simulink model "LinLongNormal_Aquila_Claws_Discrete"  (R2017a)
settings: Solver=VariableStepAuto  StartTime=0.0  StopTime=500  RelTol=1e-3  EnableMultiTasking=on
model workspace: external: MAT-File (data not in the file)
undefined symbols (not defined in the file): AP_AltLoop_AltCmdLPFDenTau, AP_AltLoop_altRateCmdMaxLimMps, AP_AltLoop_altRateCmdMinLimMps, AP_AltLoop_Kd, AP_AltLoop_Ki, AP_AltLoop_Ki_WindupMaxLim, AP_AltLoop_Ki_WindupMinLim, AP_AltLoop_Kp, AP_ClimbRate_LPFDenTau, AP_ClimbRateLoop_ClimbRateCmdLPFDenTau, AP_ClimbRateLoop_Ki, AP_ClimbRateLoop_Kp, AP_ClimbRateLoop_LLFiltDenCoe, AP_ClimbRateLoop_LLFiltNumCoe, AP_ClimbRateLoop_MaxPitchCmdrad, AP_ClimbRateLoop_MinPitchCmdrad, AP_FlexLoop_NotchDampingDen, AP_FlexLoop_NotchDampingNum, AP_FlexLoop_NotchFreq, AP_FlexLoop_nzFdbk_Kp, AP_FlexLoop_nzFdbkLLFiltDenCoe, AP_FlexLoop_nzFdbkLLFiltNumCoe, AP_FlexLoop_wn_ElvRollOff, AP_GLALoop_MaxSplCmdDeg, AP_GLALoop_MinSplCmdDeg, AP_GLALoop_nzFdbk_Ki, AP_GLALoop_nzFdbk_Kp, AP_GLALoop_nzFdbkDenTau, AP_GndTrkLoop_CmdLPFDenTau, AP_GndTrkLoop_Kd, AP_GndTrkLoop_Kp, AP_GndTrkLoop_phiCmdMaxLimDeg, AP_GndTrkLoop_phiCmdMinLimDeg, AP_GndTrkLoop_phiRateCmdMaxLimDps, AP_GndTrkLoop_phiRateCmdMinLimDps, AP_PitchLoop_DerivLPFDenTau, AP_PitchLoop_Kd, AP_PitchLoop_Kff, AP_PitchLoop_Ki, AP_PitchLoop_Kp, AP_PitchLoop_Kq, AP_PitchLoop_Notch1BWfactor, AP_PitchLoop_Notch1CosFreqNorm, AP_PitchLoop_qFdbkLFLLFiltDenCoe, AP_PitchLoop_qFdbkLFLLFiltNumCoe, AP_PitchLoop_qFdbkLLFiltDenCoe, AP_PitchLoop_qFdbkLLFiltNumCoe, AP_PitchLoop_thetaCmdLPFDenTau, AP_PitchLoop_wn_ElvRollOff, AP_PitchLoop_zeta_ElvRollOff, AP_PwrLoop_ClimbRateCmdLPFDenTau, AP_PwrLoop_Ki, AP_PwrLoop_Kp, AP_PwrLoop_Kvadv, AP_PwrLoop_LLFiltDenCoe, AP_PwrLoop_LLFiltNumCoe, AP_PwrLoop_MaxThrCmdNorm, AP_PwrLoop_MinThrCmdNorm, AP_PwrLoop_wn_ThrRollOff, AP_PwrLoop_zeta_ThrRollOff ... (+59)
libraries: discretizing x18, aerolibconvert2 x15, simulink x10, Washout x1, cstblocks x1
(part 1 of 2)
settings Model: Creator=The MathWorks, Inc.  LastModifiedBy=hbolandhemmat
settings DataIOCC: LimitDataPoints=on
settings OptimizationCC: LifeSpan=inf
settings DebuggingCC: AllowSymbolicDim=off  SFUnexpectedBacktrackingDiag=warning  SFNoUnconditionalDefaultTransitionDiag=warning  SFExecutionAtInitializationDiag=none
settings ModelReferenceCC: PropagateSignalLabelsOutOfModel=off
settings GRTTargetCC: TargetLangStandard=C89/C90 (ANSI)
settings ConfigComp: CovMetricSettings=dw  CovHtmlReporting=on  CovSaveCumulativeToWorkspaceVar=on  CovSaveSingleToWorkspaceVar=on  CovExternalEMLEnable=off

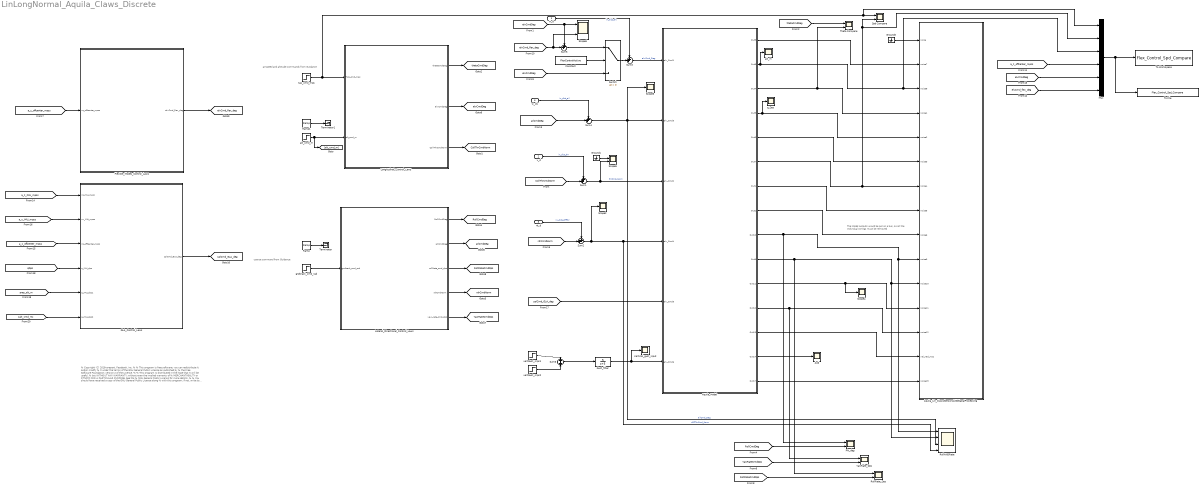
== system LinLongNormal_Aquila_Claws_Discrete ==
  note: coarse command from Guidance
  note: The Model outputs would be put on a bus, so all
      | the individual strings must be removed
  note: airspeed and altitude commands
      | from Guidance
  note: % Copyright (C) 2018-present, Facebook, Inc.
      | %
      | % This program is free software; you can redistribute it and/or modify
      | % it under the terms of the GNU General Public License as published by
      | % the Free Software Foundation; version 2 of the License.
      | %
      | % This program is distributed in the hope that it will be useful,
      | % but WITHOUT ANY WARRANTY; without even the implied warranty of
      | % MERCHANTABILITY or FITNESS FOR A PARTICULAR PURPOSE. See the
      | % GNU General Public License for more details.
      | %
      | % You should have received a copy of the GNU General Public License along
      | % with this program; if not, write to the Free Software Foundation, Inc.,
      | % 51 Franklin Street, Fifth Floor, Boston, MA 02110-1301 USA.
  w_d : Inport
  v_d : Inport  Port=2
  nt_d : Inport  Port=3
  w_d1 : Inport  Port=4
  AoS : Scope
  Aquila_Lin_ClawsSensorsANDSignalProcessing : Subsystem
  Aquila_Model : Subsystem
  Constant : Constant  Value=FlexControlActive
  Flexible_Modes_Control_Laws : Subsystem
  GLA_Control_Laws : Subsystem
  Ground1 : Ground
  Ground3 : Ground
  Gust_filter : TransferFcn  Numerator=[5]  Denominator=[1 5]
  Lateral_Directional_Control_Laws : Subsystem
  Longitudinal_Control_Laws : Subsystem
  Mux : Mux  Inputs=6
  Phi_deg : Scope  NumInputPorts=2
  Ramp : simulink/Sources/Ramp  slope=0.02  start=1  X0=0
  Ramp1 : simulink/Sources/Ramp  slope=0.35  start=1  X0=0
  RollANDRate : Scope  NumInputPorts=4
  RollRate_Dps : Scope  NumInputPorts=2
  Scope2 : Scope
  Scope3 : Scope
  Scope4 : Scope
  Scope5 : Scope  NumInputPorts=2
  Scope6 : Scope  NumInputPorts=2
  Spd Compare : Scope  NumInputPorts=2
  Sum{1..5} (5 alike) : Sum  Inputs=++|
  Sum6 : Sum  Inputs=+|+
  Switch : Switch  Criteria=u2 > Threshold
  Terminator : Terminator
  Terminator1 : Terminator
  Theta Compare : Scope  NumInputPorts=2
  To File : ToFile  Filename=Flex_Control_Spd_Compare  MatrixName=Flex_Control_Spd_Compare_dataset  SaveFormat=Timeseries
  To Workspace : ToWorkspace  VariableName=Flex_Control_Spd_Compare  SaveFormat=Timeseries  SampleTime=-1
  Vertical_gust_input : Scope
  YawRate_Dps : Scope  NumInputPorts=2
  alt_cmd_m : Step  After=0  SampleTime=0
  alt_m : Scope
  gndtrack_cmd_rad : Step  After=0  SampleTime=0
  q_Dps : Scope
  tas_cmd_mps : Step  After=10  SampleTime=0
  vertGust_mps1 : Step  Time=5  After=0  SampleTime=0
  vertGust_mps2 : Step  Time=9  After=0  SampleTime=0
  tag scope: CollThrCmdNorm=global, RollCmdDeg=global, RollRateCmdDps=global, YawRateCmdDps=global, ailCmdDeg=global, elvCmdDeg=global, elvCmd_flex_deg=global, rdrCmdNorm=global, splCmd_GLA_deg=global, thetaCmdDeg=global
  wires:
  w_d/1 -> Sum3/1  "in_dist_elv"
  Sum3/1 -> Aquila_Model/1(elv_Cmd1)  "elvCmd_Deg"
  Ground3/1 -> Aquila_Lin_ClawsSensorsANDSignalProcessing/1(noise)
  Aquila_Model/4(Out5) -> q_Dps/1, Aquila_Lin_ClawsSensorsANDSignalProcessing/5(noise2)
  Aquila_Model/3(Out4) -> Aquila_Lin_ClawsSensorsANDSignalProcessing/4(noise1), Theta Compare/2
  Aquila_Model/1(Out3) -> Aquila_Lin_ClawsSensorsANDSignalProcessing/2(noise7)
  Aquila_Model/7(Out1) -> Aquila_Lin_ClawsSensorsANDSignalProcessing/8(noise5)
  Aquila_Model/8(Out2) -> Aquila_Lin_ClawsSensorsANDSignalProcessing/9(noise6)
  Aquila_Model/2(Out8) -> Mux/3, Aquila_Lin_ClawsSensorsANDSignalProcessing/3(noise8), alt_m/1
  v_d/1 -> Sum1/1  "in_dist_thr"
  Sum1/1 -> Aquila_Model/3(elv_Cmd2), Scope5/2  "thrCmd_Norm"
  Aquila_Model/5(Out6) -> Aquila_Lin_ClawsSensorsANDSignalProcessing/6(noise3)
  alt_cmd_m/1 -> Longitudinal_Control_Laws/2(alt_cmd_m), [alt_cmd_m]
  Ground1/1 -> Scope5/1
  Longitudinal_Control_Laws/2(elvCmdDeg) -> [elvCmdDeg]
  Longitudinal_Control_Laws/3(CollThrCmdNorm) -> [CollThrCmdNorm]
  [CollThrCmdNorm] -> Sum1/2
  [elvCmdDeg] -> Sum5/1, Scope6/1
  Longitudinal_Control_Laws/1(thetaCmdDeg) -> [thetaCmdDeg]
  [thetaCmdDeg] -> Theta Compare/1
  gndtrack_cmd_rad/1 -> Lateral_Directional_Control_Laws/1(gndtrack_cmd_rad)
  Lateral_Directional_Control_Laws/2(ailCmdDeg) -> [ailCmdDeg]
  Lateral_Directional_Control_Laws/1(RollCmdDeg) -> [RollCmdDeg]
  Aquila_Model/9(Out10) -> Phi_deg/1, Aquila_Lin_ClawsSensorsANDSignalProcessing/10(noise9), RollANDRate/1
  Aquila_Model/10(Out9) -> RollRate_Dps/1, RollANDRate/2, Aquila_Lin_ClawsSensorsANDSignalProcessing/11(noise10)
  Aquila_Model/11(Out11) -> Scope4/1, Aquila_Lin_ClawsSensorsANDSignalProcessing/12(noise11)
  Aquila_Model/12(Out12) -> YawRate_Dps/1, Aquila_Lin_ClawsSensorsANDSignalProcessing/13(noise12)
  [RollCmdDeg] -> Phi_deg/2
  Aquila_Model/13(Out13) -> Aquila_Lin_ClawsSensorsANDSignalProcessing/14(vel_ned_mps)
  Lateral_Directional_Control_Laws/4(rdrCmdNorm) -> [rdrCmdNorm]
  Sum2/1 -> Scope2/1, RollANDRate/4, Aquila_Model/4(elv_Cmd4)  "diffThrCmd_Norm"
  nt_d/1 -> Sum2/1  "in_dist_diffthr"
  Lateral_Directional_Control_Laws/5(yaw_rate_cmd_dps) -> [YawRateCmdDps]
  [YawRateCmdDps] -> YawRate_Dps/2
  [RollRateCmdDps] -> RollRate_Dps/2
  Lateral_Directional_Control_Laws/3(rollRate_cmd_dps) -> [RollRateCmdDps]
  Aquila_Model/14(Out14) -> AoS/1
  Ramp/1 -> Terminator/1
  w_d1/1 -> Sum4/1  "in_dist_ail"
  Sum4/1 -> RollANDRate/3, Aquila_Model/2(elv_Cmd3), Scope3/1  "ailCmd_Deg"
  [splCmd_GLA_deg] -> Aquila_Model/5(elv_Cmd5)
  Ramp1/1 -> Terminator1/1
  [a_z_offcenter_mpss] -> Flexible_Modes_Control_Laws/1(nz_offcenter_mpss)
  Flexible_Modes_Control_Laws/1(elvCmd_flex_deg) -> [elvCmd_flex_deg]
  [elvCmd_flex_deg] -> Scope6/2, Sum5/2
  [ailCmdDeg] -> Sum4/2
  [rdrCmdNorm] -> Sum2/2
  tas_cmd_mps/1 -> Mux/1, Spd Compare/1, Longitudinal_Control_Laws/1(TAS_cmd_mps)
  Aquila_Model/6(Out7) -> Mux/2, Spd Compare/2, Aquila_Lin_ClawsSensorsANDSignalProcessing/7(noise4)
  [a_z_offcenter_mpss] -> Mux/4
  [elvCmd_flex_deg] -> Mux/6
  [elvCmdDeg] -> Mux/5
  Mux/1 -> To File/1, To Workspace/1
  Constant/1 -> Switch/2
  [elvCmdDeg] -> Switch/3
  Switch/1 -> Sum3/2
  Sum5/1 -> Switch/1
  vertGust_mps2/1 -> Sum6/2
  vertGust_mps1/1 -> Sum6/1
  Sum6/1 -> Gust_filter/1
  GLA_Control_Laws/1(splCmd_GLA_deg) -> [splCmd_GLA_deg]
  [a_z_IMU_mpss] -> GLA_Control_Laws/1(nz_IMU_mpss)
  [a_x_IMU_mpss] -> GLA_Control_Laws/2(nx_IMU_mpss)
  [a_z_offcenter_mpss] -> GLA_Control_Laws/3(nz_offcenter_mpss)
  Gust_filter/1 -> Vertical_gust_input/1, Aquila_Model/6(elv_Cmd6)
  [qDps] -> GLA_Control_Laws/4(q_IMU_dps)
  [pres_alt_m] -> GLA_Control_Laws/5(q_IMU_dps1)
  [alt_cmd_m] -> GLA_Control_Laws/6(q_IMU_dps2)
  Aquila_Model/15(Out17) -> Aquila_Lin_ClawsSensorsANDSignalProcessing/15(noise15)

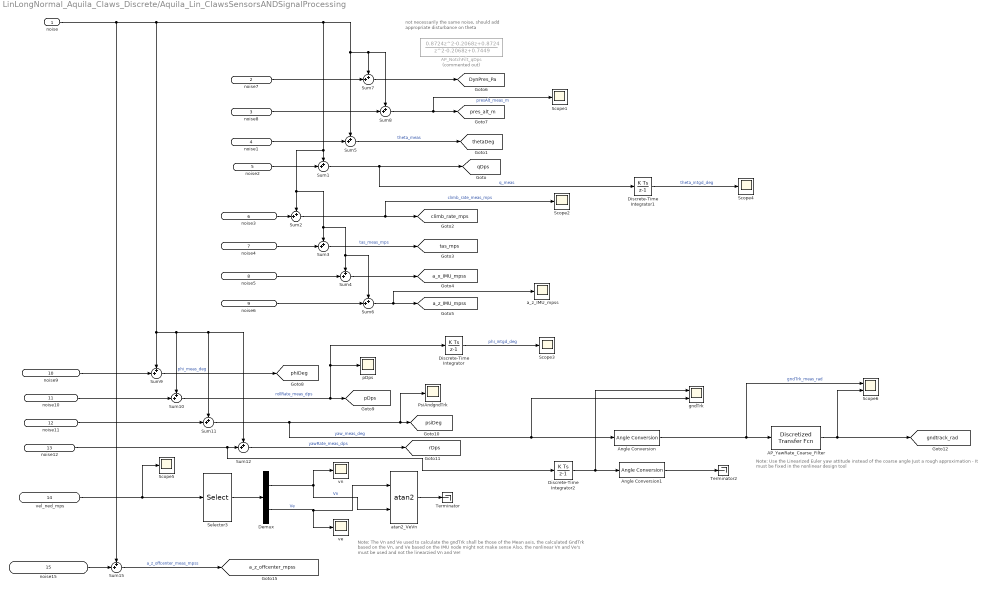
== system LinLongNormal_Aquila_Claws_Discrete/Aquila_Lin_ClawsSensorsANDSignalProcessing ==
  note: Note: The Vn and Ve used to calculate the gndTrk shall be those of the Mean axis, the
      | calculated GndTrk based on the Vn, and Ve based on the IMU node might not make sense
      |
      | Also, the nonlinear Vn and Ve's must be used and not the linearzied Vn and Ve!
  note: not necessarily the same noise,
      | should add appropriate disturbance on theta
  note: Note: Use the Linearized Euler yaw attitude instead of the coarse angle
      | Just a rough approximation - It must be fixed in the nonlinear design tool
  noise : Inport
  noise7 : Inport  Port=2
  noise8 : Inport  Port=3
  noise1 : Inport  Port=4
  noise2 : Inport  Port=5
  noise3 : Inport  Port=6
  noise4 : Inport  Port=7
  noise5 : Inport  Port=8
  noise6 : Inport  Port=9
  noise9 : Inport  Port=10
  noise10 : Inport  Port=11
  noise11 : Inport  Port=12
  noise12 : Inport  Port=13
  vel_ned_mps : Inport  Port=14
  noise15 : Inport  Port=15
  AP_NotchFilt_qDps : DiscreteTransferFcn  Commented=on  Numerator=[0.8724 -0.2068 0.8724]  Denominator=[1 -0.2068 0.7449]  SampleTime=Ts
  AP_YawRate_Coarse_Filter : discretizing/Discretized Transfer Fcn  Numerator=[1]  Denominator=[1 1]  AbsTol=auto  SampleTime=Ts  method=zoh  Wc=1
  Angle Conversion : aerolibconvert2/Angle Conversion  IU=deg  OU=rad
  Angle Conversion1 : aerolibconvert2/Angle Conversion  IU=deg  OU=rad
  Demux : Demux  Outputs=2
  Discrete-Time Integrator : DiscreteIntegrator  gainval=1  InitialConditionSetting=State (most efficient)  SampleTime=-1  ICPrevOutput=DiscIntNeverNeededParam  ICPrevScaledInput=DiscIntNeverNeededParam
  Discrete-Time Integrator1 : DiscreteIntegrator  gainval=1  InitialConditionSetting=State (most efficient)  SampleTime=-1  ICPrevOutput=DiscIntNeverNeededParam  ICPrevScaledInput=DiscIntNeverNeededParam
  Discrete-Time Integrator2 : DiscreteIntegrator  gainval=1  InitialConditionSetting=State (most efficient)  SampleTime=Ts  ICPrevOutput=DiscIntNeverNeededParam  ICPrevScaledInput=DiscIntNeverNeededParam
  PsiAndgndTrk : Scope
  Scope{1..5} (5 alike) : Scope
  Scope6 : Scope  NumInputPorts=2
  Selector3 : Selector  InputPortWidth=3  IndexOptions=Index vector (dialog)  Indices=1:2  OutputSizes=1
  Sum{1..12,15} (13 alike) : Sum  Inputs=++|
  Terminator : Terminator
  Terminator2 : Terminator
  a_z_IMU_mpss : Scope
  atan2_VeVn : Trigonometry  Operator=atan2
  gndTrk : Scope  NumInputPorts=2
  pDps : Scope
  ve : Scope
  vn : Scope
  tag scope: DynPres_Pa=global, a_x_IMU_mpss=global, a_z_IMU_mpss=global, a_z_offcenter_mpss=global, climb_rate_mps=global, gndtrack_rad=global, pDps=global, phiDeg=global, pres_alt_m=global, psiDeg=global, qDps=global, rDps=global, tas_mps=global, thetaDeg=global
  wires:
  noise1/1 -> Sum5/2
  noise2/1 -> Sum1/2
  Sum5/1 -> [thetaDeg]  "theta_meas"
  Sum1/1 -> Discrete-Time Integrator1/1, [qDps]  "q_meas"
  noise3/1 -> Sum2/2
  Sum2/1 -> Scope2/1, [climb_rate_mps]  "climb_rate_meas_mps"
  noise4/1 -> Sum3/2
  Sum3/1 -> [tas_mps]  "tas_meas_mps"
  noise5/1 -> Sum4/2
  Sum4/1 -> [a_x_IMU_mpss]
  noise6/1 -> Sum6/2
  Sum6/1 -> a_z_IMU_mpss/1, [a_z_IMU_mpss]
  noise7/1 -> Sum7/2
  Sum7/1 -> [DynPres_Pa]
  noise8/1 -> Sum8/2
  Sum8/1 -> Scope1/1, [pres_alt_m]  "presAlt_meas_m"
  noise9/1 -> Sum9/2
  noise10/1 -> Sum10/2
  noise12/1 -> Discrete-Time Integrator2/1, Sum12/2
  noise11/1 -> Sum11/2
  Sum9/1 -> [phiDeg]  "phi_meas_deg"
  Sum10/1 -> Discrete-Time Integrator/1, pDps/1, [pDps]  "rollRate_meas_dps"
  Sum11/1 -> PsiAndgndTrk/1, [psiDeg], gndTrk/2, Angle Conversion/1  "yaw_meas_deg"
  Sum12/1 -> [rDps]  "yawRate_meas_dps"
  Selector3/1 -> Demux/1
  Demux/2 -> atan2_VeVn/1, ve/1  "Ve"
  Demux/1 -> atan2_VeVn/2, vn/1  "Vn"
  vel_ned_mps/1 -> Scope5/1, Selector3/1
  Discrete-Time Integrator/1 -> Scope3/1  "phi_intgd_deg"
  Discrete-Time Integrator1/1 -> Scope4/1  "theta_intgd_deg"
  noise15/1 -> Sum15/2
  noise/1 -> Sum12/1, Sum11/1, Sum10/1, Sum9/1, Sum5/1, Sum8/1, Sum7/1, Sum6/1, Sum4/1, Sum3/1, Sum2/1, Sum1/1, Sum15/1
  Sum15/1 -> [a_z_offcenter_mpss]  "a_z_offcenter_meas_mpss"
  atan2_VeVn/1 -> Terminator/1
  Angle Conversion/1 -> Scope6/1, AP_YawRate_Coarse_Filter/1  "gndTrk_meas_rad"
  Discrete-Time Integrator2/1 -> gndTrk/1, Angle Conversion1/1
  Angle Conversion1/1 -> Terminator2/1
  AP_YawRate_Coarse_Filter/1 -> Scope6/2, [gndtrack_rad]

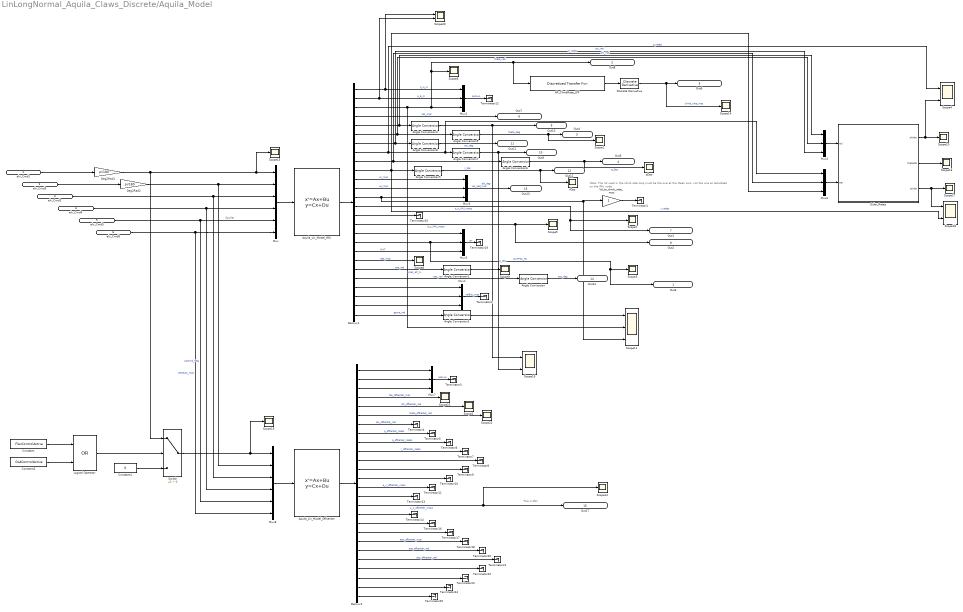
== system LinLongNormal_Aquila_Claws_Discrete/Aquila_Model ==
  note: Spoiler
  note: Note: The Vd used in the climb rate loop must be the one at the Mean axis,
      | not the one at calculated on the IMU node
  note: This is dNz
  elv_Cmd1 : Inport
  elv_Cmd3 : Inport  Port=2
  elv_Cmd2 : Inport  Port=3
  elv_Cmd4 : Inport  Port=4
  elv_Cmd5 : Inport  Port=5
  elv_Cmd6 : Inport  Port=6
  AP_ClimbRate_LPF : discretizing/Discretized Transfer Fcn  Numerator=[1]  Denominator=[AP_ClimbRate_LPFDenTau 1]  AbsTol=auto  SampleTime=Ts  method=zoh  Wc=1
  Angle Conversion{,1..3,5..9} (9 alike) : aerolibconvert2/Angle Conversion  IU=rad  OU=deg
  Aquila_Lin_Model_IMU : StateSpace  A=LIN_AC_S_A  B=LIN_AC_S_B  C=LIN_AC_S_C  D=LIN_AC_S_D  X0=0
  Aquila_Lin_Model_Offcenter : StateSpace  A=LIN_FLEX_AC_S_A  B=LIN_FLEX_AC_S_B  C=LIN_FLEX_AC_S_C  D=LIN_FLEX_AC_S_D  X0=0
  Constant : Constant  Value=FlexControlActive
  Constant1 : Constant  Value=0
  Constant2 : Constant  Value=GLAControlActive
  Deg2Rad1 : Gain  Gain=pi/180
  Deg2Rad2 : Gain  Gain=pi/180
  Demux1 : Demux  Outputs=26
  Demux2 : Demux  Outputs=26
  Discrete Derivative : simulink/Discrete/Discrete Derivative  gainval=1.0  ICPrevScaledInput=0.0  OutMin=[]  OutMax=[]  OutDataType=fixdt(1, 16)  OutScaling=2^-10  DoSatur=off
  Euler_Rates : Subsystem
  Logical Operator : Logic  Operator=OR  AllPortsSameDT=off  OutDataTypeStr=boolean
  Mux : Mux  Inputs=6
  Mux{1..7} (7 alike) : Mux  Inputs=3
  Mux8 : Mux  Inputs=6
  Scope{1..3,5..10,12..15,17,19,21..22} (17 alike) : Scope
  Scope11 : Scope  NumInputPorts=3
  Scope{4,16,18,20} (4 alike) : Scope  NumInputPorts=2
  Switch : Switch  Criteria=u2 > Threshold
  Terminator{1..25} (25 alike) : Terminator
  Vd_to_climb_rate_mps : Gain
  qDps : Scope
  rDps : Scope
  Out3 : Outport
  Out8 : Outport  Port=2
  Out4 : Outport  Port=3
  Out5 : Outport  Port=4
  Out6 : Outport  Port=5
  Out7 : Outport  Port=6
  Out1 : Outport  Port=7
  Out2 : Outport  Port=8
  Out10 : Outport  Port=9
  Out9 : Outport  Port=10
  Out11 : Outport  Port=11
  Out12 : Outport  Port=12
  Out13 : Outport  Port=13
  Out14 : Outport  Port=14
  Out17 : Outport  Port=15
  wires:
  Mux/1 -> Aquila_Lin_Model_IMU/1
  elv_Cmd1/1 -> Deg2Rad1/1
  Demux1/8 -> Scope4/1, Mux6/1, Angle Conversion7/1  "p_radps"
  Demux1/15 -> Terminator15/1
  Demux1/3 -> Scope6/1, AP_ClimbRate_LPF/1, Out8/1, Mux2/3, Scope11/2  "pres_alt_m"
  Mux2/1 -> Terminator12/1  "posLLA"
  Demux1/2 -> Mux2/2, Scope20/2  "p_E_m"
  Demux1/18 -> Out3/1, Scope3/1, Mux5/2  "DynPres_Pa"
  Demux1/17 -> Mux5/1
  Demux1/1 -> Scope20/1, Mux2/1  "p_N_m"
  Demux1/19 -> Mux5/3  "OAT"
  Mux5/1 -> Terminator19/1  "air"
  Demux1/5 -> Mux4/1, Angle Conversion3/1  "phi_rad"
  Demux1/14 -> Out1/1, Scope7/1  "a_x_IMU_mpss"
  Demux1/16 -> Out2/1, Scope5/1  "a_z_IMU_mpss"
  Demux1/7 -> Mux4/3, Angle Conversion8/1  "psi_rad"
  Demux1/6 -> Mux4/2, Angle Conversion9/1  "theta_rad"
  Angle Conversion9/1 -> Scope1/1, Out4/1  "theta_Deg"
  Demux1/9 -> Mux6/2, Angle Conversion6/1  "q_radps"
  Angle Conversion6/1 -> qDps/1, Out5/1  "q_Dps"
  Aquila_Lin_Model_IMU/1 -> Demux1/1
  Demux1/4 -> Out7/1  "tas_mps"
  Vd_to_climb_rate_mps/1 -> Terminator1/1
  Demux1/20 -> Scope8/1  "eas_mps"
  Demux1/21 -> Angle Conversion1/1  "aoa_rad"
  Demux1/22 -> Angle Conversion/1  "aos_rad"
  Demux1/23 -> Mux1/1
  Demux1/24 -> Mux1/2
  Demux1/26 -> Angle Conversion2/1  "gama_rad"
  Angle Conversion/1 -> Out14/1  "aos_deg"
  Angle Conversion1/1 -> Scope9/1
  Angle Conversion2/1 -> Scope11/1
  AP_ClimbRate_LPF/1 -> Discrete Derivative/1
  Discrete Derivative/1 -> Scope14/1, Out6/1  "climb_rate_mps"
  Demux1/10 -> Scope18/2, Mux6/3, Angle Conversion5/1  "r_radps"
  Angle Conversion5/1 -> rDps/1, Out12/1  "r_dps"
  Angle Conversion7/1 -> Scope16/2, Out9/1  "p_dps"
  Angle Conversion3/1 -> Scope16/1, Out10/1  "phi_deg"
  Angle Conversion8/1 -> Out11/1  "psi_deg"
  Mux1/1 -> Terminator2/1  "velBdy_mps"
  Demux1/25 -> Mux1/3
  Demux1/11 -> Mux3/1  "vn_mps"
  Demux1/12 -> Mux3/2  "ve_mps"
  Demux1/13 -> Scope11/3, Vd_to_climb_rate_mps/1, Mux3/3
  Mux3/1 -> Out13/1  "vel_ned_mps"
  Mux4/1 -> Euler_Rates/1(eul)
  Mux6/1 -> Euler_Rates/2(pqr)
  Euler_Rates/1(phidot) -> Scope4/2, Scope10/1
  Euler_Rates/2(thetadot) -> Scope13/1
  Euler_Rates/3(psidot) -> Scope18/1, Scope17/1
  elv_Cmd5/1 -> Mux8/5, Mux/5  "splCmd_Deg"
  elv_Cmd3/1 -> Deg2Rad2/1
  Switch/1 -> Scope19/1, Mux8/1
  Constant1/1 -> Switch/3
  elv_Cmd6/1 -> Mux8/6, Mux/6  "vertGust_mps"
  Aquila_Lin_Model_Offcenter/1 -> Demux2/1
  Demux2/5 -> Scope2/1  "phi_offcenter_rad"
  Demux2/4 -> Scope21/1  "tas_offcenter_mps"
  Demux2/21 -> Terminator20/1  "aoa_offcenter_rad"
  Demux2/15 -> Terminator13/1
  Demux2/10 -> Terminator7/1  "r_offcenter_radps"
  Demux2/1 -> Mux7/1
  Demux2/2 -> Mux7/2
  Demux2/8 -> Terminator5/1  "p_offcenter_radps"
  Demux2/7 -> Terminator4/1  "psi_offcenter_rad"
  Demux2/18 -> Terminator16/1
  Demux2/26 -> Terminator25/1
  Demux2/6 -> Scope22/1  "theta_offcenter_rad"
  Demux2/3 -> Mux7/3
  Demux2/12 -> Terminator9/1
  Demux2/13 -> Terminator10/1
  Demux2/17 -> Terminator14/1
  Demux2/20 -> Terminator18/1  "eas_offcenter_mps"
  Demux2/24 -> Terminator23/1
  Demux2/11 -> Terminator8/1
  Demux2/25 -> Terminator24/1
  Demux2/22 -> Terminator21/1  "aos_offcenter_rad"
  Demux2/16 -> Out17/1, Scope12/1  "a_z_offcenter_mpss"
  Demux2/9 -> Terminator6/1  "q_offcenter_radps"
  Demux2/14 -> Terminator11/1  "a_x_offcenter_mpss"
  Demux2/19 -> Terminator17/1
  Demux2/23 -> Terminator22/1
  Mux7/1 -> Terminator3/1  "posLLA"
  Mux8/1 -> Aquila_Lin_Model_Offcenter/1
  Deg2Rad1/1 -> Scope15/1, Mux/1, Switch/1
  Deg2Rad2/1 -> Mux8/2, Mux/2
  elv_Cmd2/1 -> Mux8/3, Mux/3
  elv_Cmd4/1 -> Mux8/4, Mux/4
  Logical Operator/1 -> Switch/2
  Constant/1 -> Logical Operator/1
  Constant2/1 -> Logical Operator/2

== system LinLongNormal_Aquila_Claws_Discrete/Flexible_Modes_Control_Laws ==
  note: Note that the Flex control loop must have a higher sampling rate than 25Hz
  note: AP_FlexLoop_Lead
  note: Aquila Aircraft Claws
      | Flexible mode control
      | Facebook Confidential
  nz_offcenter_mpss : Inport
  AP_FlexLoop_Lag : TransferFcn  Numerator=[AP_FlexLoop_wn_ElvRollOff]  Denominator=[1 AP_FlexLoop_wn_ElvRollOff]
  AP_FlexLoop_Notch : TransferFcn  Numerator=[1 2*(AP_FlexLoop_NotchDampingNum)*(AP_FlexLoop_NotchFreq) (AP_FlexLoop_NotchFreq)^2]  Denominator=[1 2*(AP_FlexLoop_NotchDampingDen)*(AP_FlexLoop_NotchFreq) (AP_FlexLoop_NotchFreq)^2]
  AP_FlexLoop_nzFdbk_Kp : Gain  Gain=AP_FlexLoop_nzFdbk_Kp
  Angle Conversion : aerolibconvert2/Angle Conversion  IU=rad  OU=deg
  Constant : Constant  Value=FlexControlActive
  Constant1 : Constant  Value=0
  OffcenterNz_Elevator : Scope  NumInputPorts=2
  Subsystem1 : Subsystem
  Switch : Switch  Criteria=u2 > Threshold
  elvCmd_flex_deg : Outport
  wires:
  nz_offcenter_mpss/1 -> AP_FlexLoop_nzFdbk_Kp/1, OffcenterNz_Elevator/1
  Angle Conversion/1 -> Switch/1, OffcenterNz_Elevator/2  "elvCmd_flex_deg"
  AP_FlexLoop_nzFdbk_Kp/1 -> Subsystem1/1(u)
  Subsystem1/1(y) -> AP_FlexLoop_Notch/1
  AP_FlexLoop_Lag/1 -> Angle Conversion/1
  AP_FlexLoop_Notch/1 -> AP_FlexLoop_Lag/1
  Constant1/1 -> Switch/3
  Constant/1 -> Switch/2
  Switch/1 -> elvCmd_flex_deg/1

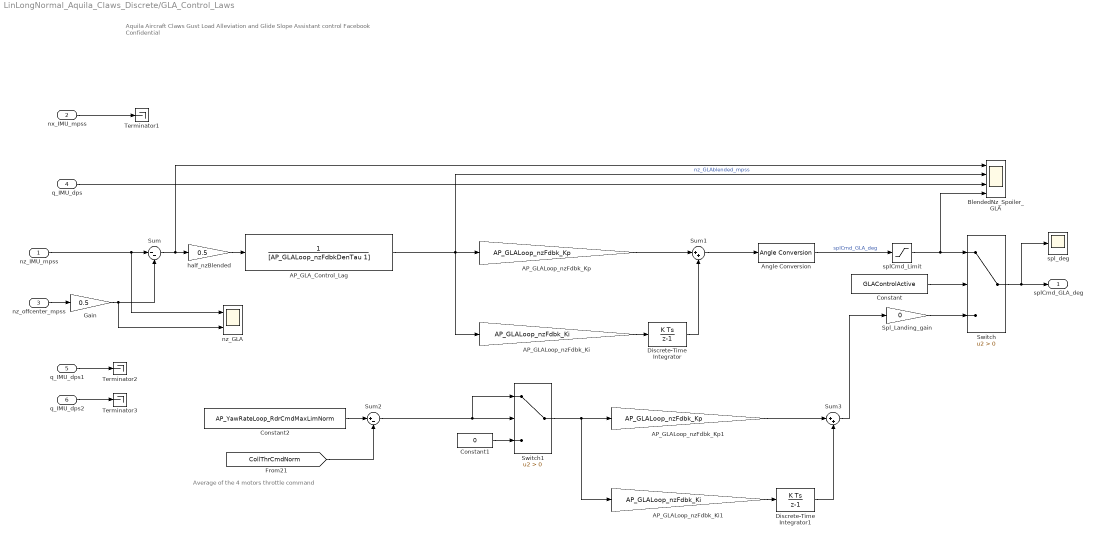
== system LinLongNormal_Aquila_Claws_Discrete/GLA_Control_Laws ==
  note: Average of the 4 motors throttle command
  note: Aquila Aircraft Claws
      | Gust Load Alleviation and Glide Slope Assistant control
      | Facebook Confidential
  nz_IMU_mpss : Inport
  nx_IMU_mpss : Inport  Port=2
  nz_offcenter_mpss : Inport  Port=3
  q_IMU_dps : Inport  Port=4
  q_IMU_dps1 : Inport  Port=5
  q_IMU_dps2 : Inport  Port=6
  AP_GLALoop_nzFdbk_Ki : Gain  Gain=AP_GLALoop_nzFdbk_Ki
  AP_GLALoop_nzFdbk_Ki1 : Gain  Gain=AP_GLALoop_nzFdbk_Ki
  AP_GLALoop_nzFdbk_Kp : Gain  Gain=AP_GLALoop_nzFdbk_Kp
  AP_GLALoop_nzFdbk_Kp1 : Gain  Gain=AP_GLALoop_nzFdbk_Kp
  AP_GLA_Control_Lag : TransferFcn  Denominator=[AP_GLALoop_nzFdbkDenTau 1]
  Angle Conversion : aerolibconvert2/Angle Conversion  IU=rad  OU=deg
  BlendedNz_Spoiler_GLA : Scope  NumInputPorts=4
  Constant : Constant  Value=GLAControlActive
  Constant1 : Constant  Value=0
  Constant2 : Constant  Value=AP_YawRateLoop_RdrCmdMaxLimNorm
  Discrete-Time Integrator : DiscreteIntegrator  InitialConditionSetting=State (most efficient)  SampleTime=-1  ICPrevOutput=DiscIntNeverNeededParam  ICPrevScaledInput=DiscIntNeverNeededParam
  Discrete-Time Integrator1 : DiscreteIntegrator  InitialConditionSetting=State (most efficient)  SampleTime=-1  ICPrevOutput=DiscIntNeverNeededParam  ICPrevScaledInput=DiscIntNeverNeededParam
  Gain : Gain  Gain=0.5
  Spl_Landing_gain : Gain  Gain=0
  Sum : Sum  Inputs=|--
  Sum1 : Sum  Inputs=|++
  Sum2 : Sum  Inputs=|+-
  Sum3 : Sum  Inputs=|++
  Switch : Switch  Criteria=u2 > Threshold
  Switch1 : Switch  Criteria=u2 > Threshold
  Terminator1 : Terminator
  Terminator2 : Terminator
  Terminator3 : Terminator
  half_nzBlended : Gain  Gain=0.5
  nz_GLA : Scope  NumInputPorts=2
  splCmd_Limit : Saturate  UpperLimit=AP_GLALoop_MaxSplCmdDeg  LowerLimit=AP_GLALoop_MinSplCmdDeg
  spl_deg : Scope
  splCmd_GLA_deg : Outport
  wires:
  Angle Conversion/1 -> splCmd_Limit/1  "splCmd_GLA_deg"
  nz_offcenter_mpss/1 -> Gain/1
  nx_IMU_mpss/1 -> Terminator1/1
  AP_GLALoop_nzFdbk_Kp/1 -> Sum1/1
  nz_IMU_mpss/1 -> nz_GLA/1, Sum/1
  AP_GLALoop_nzFdbk_Ki/1 -> Discrete-Time Integrator/1
  Discrete-Time Integrator/1 -> Sum1/2
  Sum1/1 -> Angle Conversion/1
  splCmd_Limit/1 -> Switch/1, BlendedNz_Spoiler_GLA/4
  AP_GLA_Control_Lag/1 -> AP_GLALoop_nzFdbk_Kp/1, BlendedNz_Spoiler_GLA/2, AP_GLALoop_nzFdbk_Ki/1  "nz_GLAblended_mpss"
  Sum/1 -> BlendedNz_Spoiler_GLA/1, half_nzBlended/1
  q_IMU_dps/1 -> BlendedNz_Spoiler_GLA/3
  q_IMU_dps1/1 -> Terminator2/1
  q_IMU_dps2/1 -> Terminator3/1
  Switch/1 -> spl_deg/1, splCmd_GLA_deg/1
  Constant/1 -> Switch/2
  Spl_Landing_gain/1 -> Switch/3
  Gain/1 -> nz_GLA/2, Sum/2
  half_nzBlended/1 -> AP_GLA_Control_Lag/1
  Constant2/1 -> Sum2/1
  [CollThrCmdNorm] -> Sum2/2
  Discrete-Time Integrator1/1 -> Sum3/2
  AP_GLALoop_nzFdbk_Ki1/1 -> Discrete-Time Integrator1/1
  AP_GLALoop_nzFdbk_Kp1/1 -> Sum3/1
  Sum3/1 -> Spl_Landing_gain/1
  Switch1/1 -> AP_GLALoop_nzFdbk_Ki1/1, AP_GLALoop_nzFdbk_Kp1/1
  Sum2/1 -> Switch1/1, Switch1/2
  Constant1/1 -> Switch1/3

== system LinLongNormal_Aquila_Claws_Discrete/Lateral_Directional_Control_Laws ==
  note: Aquila Aircraft Claws
      | Facebook Confidential
  gndtrack_cmd_rad : Inport
  GndTrkLoop : Subsystem
  RollLoop : Subsystem
  YawLoop : Subsystem
  RollCmdDeg : Outport
  ailCmdDeg : Outport  Port=2
  rollRate_cmd_dps : Outport  Port=3
  rdrCmdNorm : Outport  Port=4
  yaw_rate_cmd_dps : Outport  Port=5
  wires:
  gndtrack_cmd_rad/1 -> GndTrkLoop/1(alt_cmd_m)
  RollLoop/1(ail_cmd_RollRateLoop_deg) -> ailCmdDeg/1
  YawLoop/1(Rdr_cmd_YawRateLoop_norm) -> rdrCmdNorm/1
  YawLoop/2(yaw_rate_cmd_dps) -> yaw_rate_cmd_dps/1
  GndTrkLoop/1(Phi_cmd_deg) -> RollCmdDeg/1, RollLoop/1(phi_cmd_deg)
  RollLoop/3(phi_err_filt) -> YawLoop/1(alt_cmd_m)
  RollLoop/2(PhiRateCmd_Dps) -> rollRate_cmd_dps/1
  GndTrkLoop/2(PhiRate_cmd_dps) -> RollLoop/2(phiRateCmd_Dps)

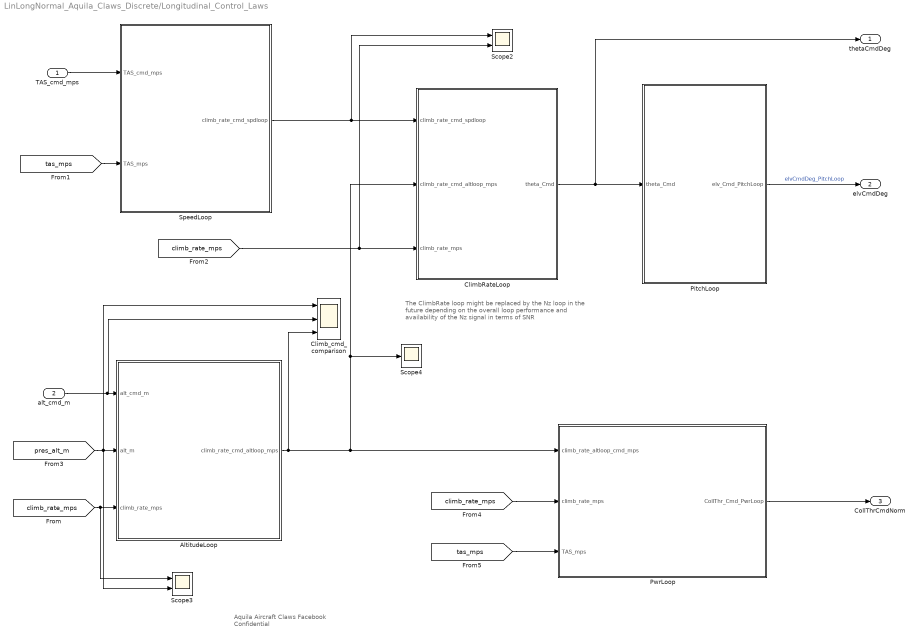
== system LinLongNormal_Aquila_Claws_Discrete/Longitudinal_Control_Laws ==
  note: Aquila Aircraft Claws
      | Facebook Confidential
  note: The ClimbRate loop might be replaced by the Nz loop
      | in the future depending on the overall loop performance
      |  and availability of the Nz signal in terms of SNR
  TAS_cmd_mps : Inport
  alt_cmd_m : Inport  Port=2
  AltitudeLoop : Subsystem
  ClimbRateLoop : Subsystem
  Climb_cmd_comparison : Scope  NumInputPorts=3
  PitchLoop : Subsystem
  PwrLoop : Subsystem
  Scope2 : Scope  NumInputPorts=2
  Scope3 : Scope  NumInputPorts=2
  Scope4 : Scope
  SpeedLoop : Subsystem
  thetaCmdDeg : Outport
  elvCmdDeg : Outport  Port=2
  CollThrCmdNorm : Outport  Port=3
  wires:
  [climb_rate_mps] -> PwrLoop/2(climb_rate_mps)
  [tas_mps] -> PwrLoop/3(TAS_mps)
  AltitudeLoop/1(climb_rate_cmd_altloop_mps) -> PwrLoop/1(climb_rate_altloop_cmd_mps), Scope4/1, ClimbRateLoop/2(climb_rate_cmd_altloop_mps), Climb_cmd_comparison/3
  PwrLoop/1(CollThr_Cmd_PwrLoop) -> CollThrCmdNorm/1
  [climb_rate_mps] -> Scope3/1, AltitudeLoop/3(climb_rate_mps)
  [pres_alt_m] -> Scope3/2, Climb_cmd_comparison/1, AltitudeLoop/2(alt_m)
  [climb_rate_mps] -> Scope2/2, ClimbRateLoop/3(climb_rate_mps)
  SpeedLoop/1(climb_rate_cmd_spdloop) -> Scope2/1, ClimbRateLoop/1(climb_rate_cmd_spdloop)
  alt_cmd_m/1 -> Climb_cmd_comparison/2, AltitudeLoop/1(alt_cmd_m)
  PitchLoop/1(elv_Cmd_PitchLoop) -> elvCmdDeg/1  "elvCmdDeg_PitchLoop"
  ClimbRateLoop/1(theta_Cmd) -> thetaCmdDeg/1, PitchLoop/1(theta_Cmd)
  [tas_mps] -> SpeedLoop/2(TAS_mps)
  TAS_cmd_mps/1 -> SpeedLoop/1(TAS_cmd_mps)

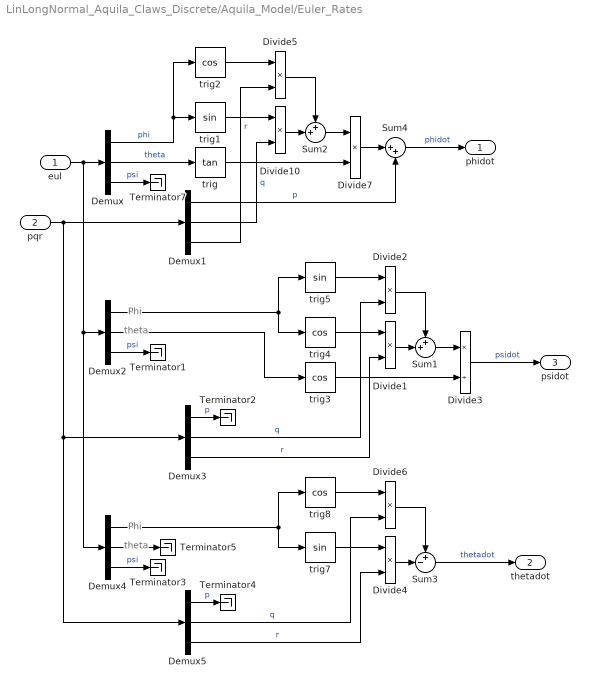
== system LinLongNormal_Aquila_Claws_Discrete/Aquila_Model/Euler_Rates ==
  note: theta
  note: Phi
  note: theta
  note: Phi
  eul : Inport
  pqr : Inport  Port=2
  Demux{,1..5} (6 alike) : Demux  Outputs=3
  Divide{1..2,4..7,10} (7 alike) : Product  Inputs=**
  Divide3 : Product  Inputs=*/
  Sum1 : Sum  Inputs=++|
  Sum2 : Sum  Inputs=++|
  Sum3 : Sum  Inputs=+-|
  Sum4 : Sum  Inputs=|++
  Terminator{1..5,7} (6 alike) : Terminator
  trig : Trigonometry  Operator=tan
  trig1 : Trigonometry
  trig{2..4,8} (4 alike) : Trigonometry  Operator=cos
  trig5 : Trigonometry
  trig7 : Trigonometry
  phidot : Outport
  thetadot : Outport  Port=2
  psidot : Outport  Port=3
  wires:
  Divide5/1 -> Sum2/1
  trig2/1 -> Divide5/1
  Divide7/1 -> Sum4/1
  Demux1/1 -> Sum4/2  "p"
  trig1/1 -> Divide10/1
  Demux1/3 -> Divide5/2  "r"
  Demux1/2 -> Divide10/2  "q"
  Sum2/1 -> Divide7/1
  trig/1 -> Divide7/2
  Sum4/1 -> phidot/1  "phidot"
  Divide10/1 -> Sum2/2
  Demux/3 -> Terminator7/1  "psi"
  Divide2/1 -> Sum1/1
  trig5/1 -> Divide2/1
  trig4/1 -> Divide1/1
  Demux/1 -> trig2/1, trig1/1  "phi"
  Demux/2 -> trig/1  "theta"
  Sum1/1 -> Divide3/1
  trig3/1 -> Divide3/2
  Divide3/1 -> psidot/1  "psidot"
  Divide1/1 -> Sum1/2
  Demux3/2 -> Divide2/2  "q"
  Demux3/3 -> Divide1/2  "r"
  Demux2/1 -> trig5/1, trig4/1
  Demux2/2 -> trig3/1
  Demux2/3 -> Terminator1/1  "psi"
  Demux3/1 -> Terminator2/1  "p"
  pqr/1 -> Demux1/1, Demux3/1, Demux5/1
  Divide6/1 -> Sum3/1
  trig8/1 -> Divide6/1
  trig7/1 -> Divide4/1
  Sum3/1 -> thetadot/1  "thetadot"
  Divide4/1 -> Sum3/2
  Demux5/2 -> Divide6/2  "q"
  Demux5/3 -> Divide4/2  "r"
  eul/1 -> Demux2/1, Demux4/1, Demux/1
  Demux4/1 -> trig8/1, trig7/1
  Demux4/3 -> Terminator3/1  "psi"
  Demux5/1 -> Terminator4/1  "p"
  Demux4/2 -> Terminator5/1

== system LinLongNormal_Aquila_Claws_Discrete/Flexible_Modes_Control_Laws/Subsystem1 ==
  u : Inport
  AP_FlexLoop_nzFdbkLLFiltDenCoe : Gain  Gain=AP_FlexLoop_nzFdbkLLFiltDenCoe
  AP_FlexLoop_nzFdbkLLFiltNumCoe : Gain  Gain=AP_FlexLoop_nzFdbkLLFiltNumCoe
  Delay : Delay  DelayLength=1  InitialCondition=0  SampleTime=Ts
  Delay1 : Delay  DelayLength=1  InitialCondition=0  SampleTime=Ts
  Sum3 : Sum  Inputs=+|+|-
  y : Outport
  wires:
  AP_FlexLoop_nzFdbkLLFiltDenCoe/1 -> Sum3/3
  u/1 -> AP_FlexLoop_nzFdbkLLFiltNumCoe/1, Sum3/1
  Delay1/1 -> AP_FlexLoop_nzFdbkLLFiltDenCoe/1
  AP_FlexLoop_nzFdbkLLFiltNumCoe/1 -> Delay/1
  Delay/1 -> Sum3/2
  Sum3/1 -> y/1, Delay1/1

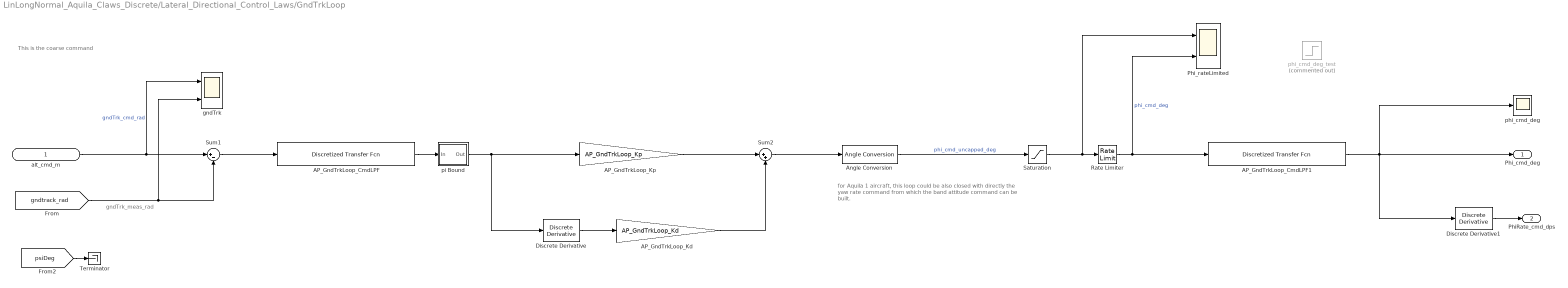
== system LinLongNormal_Aquila_Claws_Discrete/Lateral_Directional_Control_Laws/GndTrkLoop ==
  note: This is the coarse command
  note: gndTrk_meas_rad
  note: for Aquila 1 aircraft, this loop could be also closed with
      | directly the yaw rate command from which the band attitude
      | command can be built.
  alt_cmd_m : Inport
  AP_GndTrkLoop_CmdLPF : discretizing/Discretized Transfer Fcn  Numerator=[1]  Denominator=[AP_GndTrkLoop_CmdLPFDenTau 1]  AbsTol=auto  SampleTime=0.04  method=zoh  Wc=1
  AP_GndTrkLoop_CmdLPF1 : discretizing/Discretized Transfer Fcn  Numerator=[1]  Denominator=[AP_GndTrkLoop_CmdLPFDenTau 1]  AbsTol=auto  SampleTime=0.04  method=zoh  Wc=1
  AP_GndTrkLoop_Kd : Gain  Gain=AP_GndTrkLoop_Kd
  AP_GndTrkLoop_Kp : Gain  Gain=AP_GndTrkLoop_Kp
  Angle Conversion : aerolibconvert2/Angle Conversion  IU=rad  OU=deg
  Discrete Derivative : simulink/Discrete/Discrete Derivative  gainval=1.0  ICPrevScaledInput=0.0  OutMin=[]  OutMax=[]  OutDataType=fixdt(1, 16)  OutScaling=2^-10  DoSatur=off
  Discrete Derivative1 : simulink/Discrete/Discrete Derivative  gainval=1.0  ICPrevScaledInput=0.0  OutMin=[]  OutMax=[]  OutDataType=fixdt(1, 16)  OutScaling=2^-10  DoSatur=off
  Phi_rateLimited : Scope  NumInputPorts=2
  Rate Limiter : RateLimiter  RisingSlewLimit=AP_GndTrkLoop_phiRateCmdMaxLimDps  FallingSlewLimit=AP_GndTrkLoop_phiRateCmdMinLimDps  SampleTimeMode=inherited
  Saturation : Saturate  UpperLimit=AP_GndTrkLoop_phiCmdMaxLimDeg  LowerLimit=AP_GndTrkLoop_phiCmdMinLimDeg
  Sum1 : Sum  Inputs=|+-
  Sum2 : Sum  Inputs=|++
  Terminator : Terminator
  gndTrk : Scope  NumInputPorts=2
  phi_cmd_deg : Scope
  phi_cmd_deg_test : Step  Commented=on  After=5  SampleTime=0
  pi Bound : Subsystem  mask(pi bound){}
      mask help: Bounds the input angle to [-pi, pi]. When -pi bound is exceeded the output wraps back to pi; when the pi bound is exceeded the output wraps back to -pi.
      mask Help:
      | Bounds the input angle to [-pi, pi]. When -pi bound is exceeded the output wraps back to pi; when the pi bound is exceeded the output wraps back to -pi.
      | <P><B>Input:</B> any angle in radians, from -Inf to Inf;</P>
      | <P><B>Output:</B> an angle in radians between -pi and pi.</P>
  Phi_cmd_deg : Outport
  PhiRate_cmd_dps : Outport  Port=2
  wires:
  alt_cmd_m/1 -> Sum1/1, gndTrk/1  "gndTrk_cmd_rad"
  [psiDeg] -> Terminator/1
  AP_GndTrkLoop_Kp/1 -> Sum2/1
  Sum1/1 -> AP_GndTrkLoop_CmdLPF/1
  AP_GndTrkLoop_Kd/1 -> Sum2/2
  Discrete Derivative/1 -> AP_GndTrkLoop_Kd/1
  Angle Conversion/1 -> Saturation/1  "phi_cmd_uncapped_deg"
  Sum2/1 -> Angle Conversion/1
  [gndtrack_rad] -> Sum1/2, gndTrk/2
  AP_GndTrkLoop_CmdLPF/1 -> pi Bound/1(In)
  pi Bound/1(Out) -> AP_GndTrkLoop_Kp/1, Discrete Derivative/1
  Discrete Derivative1/1 -> PhiRate_cmd_dps/1
  Saturation/1 -> Phi_rateLimited/1, Rate Limiter/1
  Rate Limiter/1 -> AP_GndTrkLoop_CmdLPF1/1, Phi_rateLimited/2  "phi_cmd_deg"
  AP_GndTrkLoop_CmdLPF1/1 -> Discrete Derivative1/1, phi_cmd_deg/1, Phi_cmd_deg/1

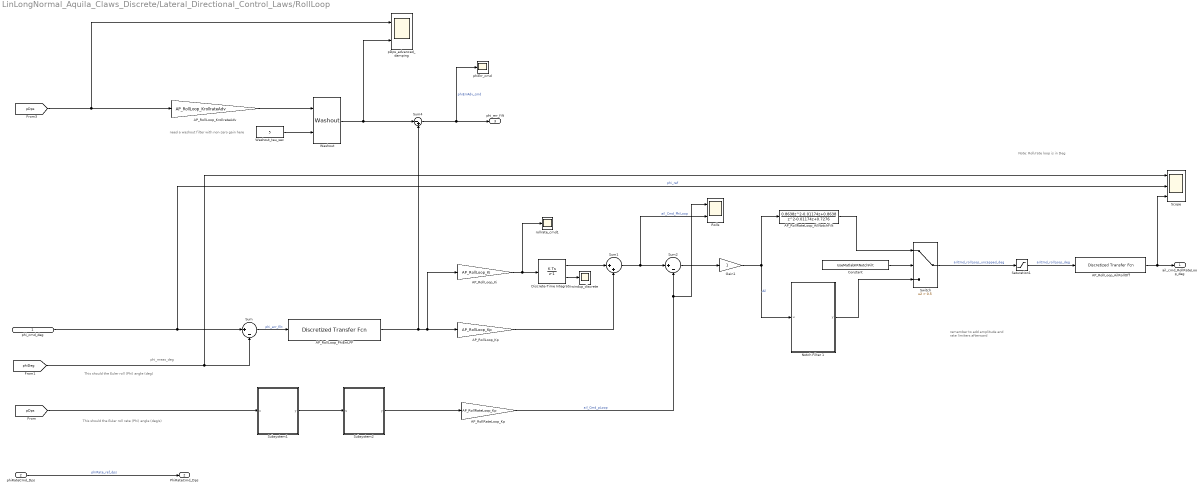
== system LinLongNormal_Aquila_Claws_Discrete/Lateral_Directional_Control_Laws/RollLoop ==
  note: need a washout filter with non-zero gain here
  note: phi_meas_deg
  note: This should the Euler roll (Phi) angle (deg)
  note: This should the Euler roll rate (Phi) angle (deg/s)
  note: remember to add amplitude and
      | rate limiters afterward
  note: Note: Roll/rate loop is in Deg
  phi_cmd_deg : Inport
  phiRateCmd_Dps : Inport  Port=2
  " pDps_advanced_damping" : Scope  NumInputPorts=2
  AP_RollLoop_AilRollOff : discretizing/Discretized Transfer Fcn  Numerator=[AP_RollLoop_wn_AilRollOff^2]  Denominator=[1 2*AP_RollLoop_zeta_AilRollOff*AP_RollLoop_wn_AilRollOff AP_RollLoop_wn_AilRollOff^2]  AbsTol=auto  SampleTime=Ts  method=zoh  Wc=1
  AP_RollLoop_Ki : Gain  Gain=AP_RollLoop_Ki
  AP_RollLoop_Kp : Gain  Gain=AP_RollLoop_Kp
  AP_RollLoop_KrollrateAdv : Gain  Gain=AP_RollLoop_KrollrateAdv
  AP_RollLoop_PhiErrLPF : discretizing/Discretized Transfer Fcn  Numerator=[1]  Denominator=[AP_RollLoop_phiErrLPFDenTau 1]  AbsTol=auto  SampleTime=0.04  method=zoh  Wc=1
  AP_RollRateLoop_AilNotchFilt : DiscreteTransferFcn  Numerator=[0.8638 -0.01174 0.8638]  Denominator=[1 -0.01174 0.7276]  SampleTime=Ts
  AP_RollRateLoop_Kp : Gain  Gain=AP_RollRateLoop_Kp
  Constant : Constant  Value=UseMatlabIIRNotchFilt
  Discrete-Time Integrator : DiscreteIntegrator  InitialConditionSetting=State (most efficient)  SampleTime=Ts  LimitOutput=on  UpperSaturationLimit=AP_RollLoop_AilWindupMaxLim  LowerSaturationLimit=AP_RollLoop_AilWindupMinLim  ShowSaturationPort=on  ICPrevOutput=DiscIntNeverNeededParam  ICPrevScaledInput=DiscIntNeverNeededParam
  Gain1 : Gain
  Notch Filter 1 : Subsystem
  Rolls : Scope  NumInputPorts=2
  Saturation1 : Saturate  UpperLimit=AP_RollLoop_ailCmdMaxLim  LowerLimit=AP_RollLoop_ailCmdMinLim
  Scope : Scope  NumInputPorts=3
  Subsystem1 : Subsystem
  Subsystem2 : Subsystem
  Sum : Sum  Inputs=|+-
  Sum1 : Sum  Inputs=|++
  Sum2 : Sum  Inputs=|+-
  Sum4 : Sum  Inputs=|-+
  Switch : Switch  Criteria=u2 > Threshold  Threshold=0.5
  Washout : Washout/Washout
  Washout_tau_sec : Constant  Value=5  SampleTime=Ts
  phiErr_cmd : Scope
  rollrate_cmd1 : Scope
  windup_discrete : Scope
  ail_cmd_RollRateLoop_deg : Outport
  PhiRateCmd_Dps : Outport  Port=2
  phi_err_filt : Outport  Port=3
  wires:
  AP_RollLoop_Ki/1 -> rollrate_cmd1/1, Discrete-Time Integrator/1
  phi_cmd_deg/1 -> Scope/2, Sum/1  "phi_ref"
  [pDps] -> Subsystem1/1(u)
  AP_RollLoop_Kp/1 -> Sum1/2
  Discrete-Time Integrator/2 -> windup_discrete/1
  Subsystem1/1(y) -> Subsystem2/1(u)
  Subsystem2/1(y) -> AP_RollRateLoop_Kp/1
  Discrete-Time Integrator/1 -> Sum1/1
  Switch/1 -> Saturation1/1  "ailCmd_rollLoop_uncapped_deg"
  Saturation1/1 -> AP_RollLoop_AilRollOff/1  "ailCmd_rollLoop_deg"
  [pDps] -> AP_RollLoop_KrollrateAdv/1, " pDps_advanced_damping"/1
  phiRateCmd_Dps/1 -> PhiRateCmd_Dps/1  "phiRate_ref_dps"
  Sum1/1 -> Rolls/2, Sum2/1  "ail_Cmd_PhiLoop"
  AP_RollRateLoop_Kp/1 -> Rolls/1, Sum2/2  "ail_Cmd_pLoop"
  Sum2/1 -> Gain1/1
  Sum4/1 -> phiErr_cmd/1, phi_err_filt/1  "phiErrAdv_cmd"
  [phiDeg] -> Scope/1, Sum/2
  Sum/1 -> AP_RollLoop_PhiErrLPF/1  "phi_err_filt"
  AP_RollLoop_PhiErrLPF/1 -> Sum4/2, AP_RollLoop_Ki/1, AP_RollLoop_Kp/1
  AP_RollRateLoop_AilNotchFilt/1 -> Switch/1
  Notch Filter 1/1(y) -> Switch/3
  Constant/1 -> Switch/2
  Gain1/1 -> Notch Filter 1/1(u), AP_RollRateLoop_AilNotchFilt/1  "Ail"
  AP_RollLoop_AilRollOff/1 -> Scope/3, ail_cmd_RollRateLoop_deg/1
  AP_RollLoop_KrollrateAdv/1 -> Washout/1
  Washout/1 -> " pDps_advanced_damping"/2, Sum4/1
  Washout_tau_sec/1 -> Washout/2

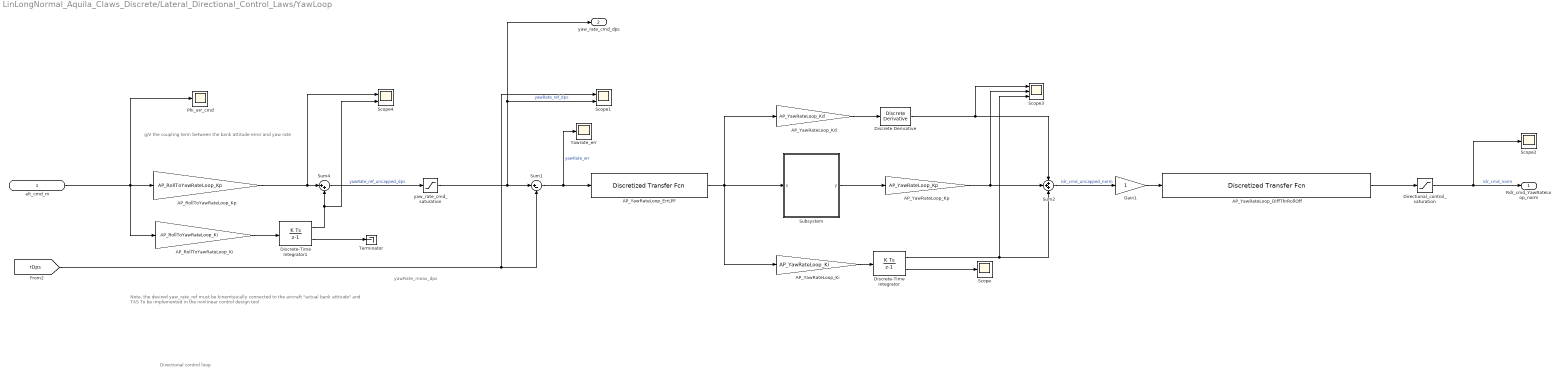
== system LinLongNormal_Aquila_Claws_Discrete/Lateral_Directional_Control_Laws/YawLoop ==
  note: yawRate_meas_dps
  note: g/V the coupling term between the bank attitude error and yaw rate
  note: Directional control loop
  note: Note, the desired yaw_rate_ref must be kinemtaically connected to the aircraft "actual bank attitude" and TAS
      | To be implemented in the nonlinear control design tool
  alt_cmd_m : Inport
  AP_RollToYawRateLoop_Ki : Gain  Gain=AP_RollToYawRateLoop_Ki
  AP_RollToYawRateLoop_Kp : Gain  Gain=AP_RollToYawRateLoop_Kp
  AP_YawRateLoop_DiffThrRollOff : discretizing/Discretized Transfer Fcn  Numerator=[AP_YawRateLoop_wn_DiffThrRollOff^2]  Denominator=[1 2*AP_YawRateLoop_zeta_DiffThrRollOff*AP_YawRateLoop_wn_DiffThrRollOff AP_YawRateLoop_wn_DiffThrRollOff^2]  AbsTol=auto  SampleTime=0.04  method=zoh  Wc=1
  AP_YawRateLoop_ErrLPF : discretizing/Discretized Transfer Fcn  Numerator=[1]  Denominator=[AP_YawRateLoop_ErrLPFDenTau 1]  AbsTol=auto  SampleTime=0.04  method=zoh  Wc=1
  AP_YawRateLoop_Kd : Gain  Gain=AP_YawRateLoop_Kd
  AP_YawRateLoop_Ki : Gain  Gain=AP_YawRateLoop_Ki
  AP_YawRateLoop_Kp : Gain  Gain=AP_YawRateLoop_Kp
  Directional_control_saturation : Saturate  UpperLimit=AP_YawRateLoop_RdrCmdMaxLimNorm  LowerLimit=AP_YawRateLoop_RdrCmdMinLimNorm
  Discrete Derivative : simulink/Discrete/Discrete Derivative  gainval=1.0  ICPrevScaledInput=0.0  OutMin=[]  OutMax=[]  OutDataType=fixdt(1, 16)  OutScaling=2^-10  DoSatur=off
  Discrete-Time Integrator : DiscreteIntegrator  InitialConditionSetting=State (most efficient)  SampleTime=-1  LimitOutput=on  UpperSaturationLimit=AP_YawRateLoop_RdrWindupMaxLim  LowerSaturationLimit=AP_YawRateLoop_RdrWindupMinLim  ShowSaturationPort=on  ICPrevOutput=DiscIntNeverNeededParam  ICPrevScaledInput=DiscIntNeverNeededParam
  Discrete-Time Integrator1 : DiscreteIntegrator  InitialConditionSetting=State (most efficient)  SampleTime=-1  LimitOutput=on  UpperSaturationLimit=AP_RollToYawRateLoop_YawRateWindupMaxLim  LowerSaturationLimit=AP_RollToYawRateLoop_YawRateWindupMinLim  ShowSaturationPort=on  ICPrevOutput=DiscIntNeverNeededParam  ICPrevScaledInput=DiscIntNeverNeededParam
  Gain1 : Gain
  Phi_err_cmd : Scope
  Scope : Scope
  Scope1 : Scope  NumInputPorts=2
  Scope2 : Scope
  Scope3 : Scope  NumInputPorts=3
  Scope4 : Scope  NumInputPorts=2
  Subsystem : Subsystem
  Sum1 : Sum  Inputs=|+-
  Sum2 : Sum  Inputs=+++
  Sum4 : Sum  Inputs=|++
  Terminator : Terminator
  Yawrate_err : Scope
  yaw_rate_cmd_saturation : Saturate  UpperLimit=AP_YawRateLoop_YawRateMaxLimDps  LowerLimit=AP_YawRateLoop_YawRateMinLimDps
  Rdr_cmd_YawRateLoop_norm : Outport
  yaw_rate_cmd_dps : Outport  Port=2
  wires:
  AP_YawRateLoop_Kp/1 -> Sum2/2, Scope3/2
  AP_YawRateLoop_Ki/1 -> Discrete-Time Integrator/1
  Directional_control_saturation/1 -> Scope2/1, Rdr_cmd_YawRateLoop_norm/1  "rdr_cmd_norm"
  Sum1/1 -> AP_YawRateLoop_ErrLPF/1, Yawrate_err/1  "yawRate_err"
  [rDps] -> Sum1/2, Scope1/1
  Sum2/1 -> Gain1/1  "rdr_cmd_uncapped_norm"
  Discrete-Time Integrator/2 -> Scope/1
  AP_YawRateLoop_Kd/1 -> Discrete Derivative/1
  Discrete-Time Integrator/1 -> Scope3/3, Sum2/3
  Discrete Derivative/1 -> Scope3/1, Sum2/1
  Gain1/1 -> AP_YawRateLoop_DiffThrRollOff/1
  alt_cmd_m/1 -> AP_RollToYawRateLoop_Ki/1, AP_RollToYawRateLoop_Kp/1, Phi_err_cmd/1
  AP_RollToYawRateLoop_Ki/1 -> Discrete-Time Integrator1/1
  Sum4/1 -> yaw_rate_cmd_saturation/1  "yawRate_ref_uncapped_dps"
  Discrete-Time Integrator1/2 -> Terminator/1
  Subsystem/1(y) -> AP_YawRateLoop_Kp/1
  AP_YawRateLoop_DiffThrRollOff/1 -> Directional_control_saturation/1
  Discrete-Time Integrator1/1 -> Scope4/2, Sum4/2
  AP_RollToYawRateLoop_Kp/1 -> Scope4/1, Sum4/1
  yaw_rate_cmd_saturation/1 -> yaw_rate_cmd_dps/1, Scope1/2, Sum1/1  "yawRate_ref_dps"
  AP_YawRateLoop_ErrLPF/1 -> AP_YawRateLoop_Ki/1, AP_YawRateLoop_Kd/1, Subsystem/1(u)

== system LinLongNormal_Aquila_Claws_Discrete/Longitudinal_Control_Laws/AltitudeLoop ==
  note: The Satuartion Block must be
      | included Later
  note: Alt loop,
      | complementary filter should be added to provide the alt_rate
  alt_cmd_m : Inport
  alt_m : Inport  Port=2
  climb_rate_mps : Inport  Port=3
  AP_AltLoop_AltCmdLPF : discretizing/Discretized Transfer Fcn  Numerator=[1]  Denominator=[AP_AltLoop_AltCmdLPFDenTau 1]  AbsTol=auto  SampleTime=Ts  method=zoh  Wc=1
  AP_AltLoop_Kd : Gain  Gain=AP_AltLoop_Kd
  AP_AltLoop_Ki : Gain  Gain=AP_AltLoop_Ki
  AP_AltLoop_Kp : Gain  Gain=AP_AltLoop_Kp
  Discrete-Time Integrator : DiscreteIntegrator  InitialConditionSetting=State (most efficient)  SampleTime=Ts  LimitOutput=on  UpperSaturationLimit=AP_AltLoop_Ki_WindupMaxLim  LowerSaturationLimit=AP_AltLoop_Ki_WindupMinLim  ShowSaturationPort=on  ICPrevOutput=DiscIntNeverNeededParam  ICPrevScaledInput=DiscIntNeverNeededParam
  Rate Limiter : RateLimiter  RisingSlewLimit=AP_AltLoop_altRateCmdMaxLimMps  FallingSlewLimit=AP_AltLoop_altRateCmdMinLimMps  SampleTimeMode=inherited
  Scope1 : Scope  NumInputPorts=4
  Scope2 : Scope  NumInputPorts=4
  Scope3 : Scope
  Scope4 : Scope
  Scope5 : Scope  NumInputPorts=2
  Sum : Sum  Inputs=|+-
  Sum1 : Sum  Inputs=+|+|-
  climb_rate_cmd_protection : Saturate  UpperLimit=AP_TASLoop_MaxClimbRateCmdmps  LowerLimit=AP_TASLoop_MinClimbRateCmdmps
  climb_rate_cmd_altloop_mps : Outport
  wires:
  AP_AltLoop_Ki/1 -> Discrete-Time Integrator/1
  Sum/1 -> AP_AltLoop_Ki/1, AP_AltLoop_Kp/1  "alt_error_m"
  AP_AltLoop_Kp/1 -> Scope1/3, Sum1/1, Scope5/1
  Discrete-Time Integrator/1 -> Sum1/2, Scope1/2, Scope5/2
  alt_cmd_m/1 -> Scope2/1, Rate Limiter/1  "alt_cmd_m"
  AP_AltLoop_AltCmdLPF/1 -> Scope2/3, Sum/1
  alt_m/1 -> Scope2/4, Sum/2
  Sum1/1 -> climb_rate_cmd_protection/1  "climb_rate_cmd_altloop_uncapped_mps"
  climb_rate_mps/1 -> AP_AltLoop_Kd/1
  AP_AltLoop_Kd/1 -> Scope1/1, Sum1/3
  climb_rate_cmd_protection/1 -> Scope1/4, Scope4/1, climb_rate_cmd_altloop_mps/1  "climb_rate_cmd_altloop_mps"
  Discrete-Time Integrator/2 -> Scope3/1
  Rate Limiter/1 -> Scope2/2, AP_AltLoop_AltCmdLPF/1

== system LinLongNormal_Aquila_Claws_Discrete/Longitudinal_Control_Laws/ClimbRateLoop ==
  note: The derivative term would consist of the delta_Nz cmd, hdd = dNz
  note: Vertical Rate loop,
      | consider taking into account the aircraft TAS when calculting the theta_cmd in case the proportional gains turned out to be large
  climb_rate_cmd_spdloop : Inport
  climb_rate_cmd_altloop_mps : Inport  Port=2
  climb_rate_mps : Inport  Port=3
  AP_ClimbRateLoop_ClimbRateCmdLPF : discretizing/Discretized Transfer Fcn  Numerator=[1]  Denominator=[AP_ClimbRateLoop_ClimbRateCmdLPFDenTau 1]  AbsTol=auto  SampleTime=0.04  method=zoh  Wc=1
  AP_ClimbRateLoop_Ki : Gain  Gain=AP_ClimbRateLoop_Ki
  AP_ClimbRateLoop_Kp : Gain  Gain=AP_ClimbRateLoop_Kp
  Angle Conversion : aerolibconvert2/Angle Conversion  IU=rad  OU=deg
  ClimbRate_cmd_compare : Scope  NumInputPorts=2
  Discrete-Time Integrator : DiscreteIntegrator  InitialConditionSetting=State (most efficient)  SampleTime=-1  LimitOutput=on  UpperSaturationLimit=0.1  LowerSaturationLimit=-0.1  ICPrevOutput=DiscIntNeverNeededParam  ICPrevScaledInput=DiscIntNeverNeededParam
  Scope : Scope
  Scope2 : Scope  NumInputPorts=3
  Subsystem : Subsystem
  Sum : Sum  Inputs=|+-
  Sum1 : Sum  Inputs=++|
  Terminator : Terminator
  pitch_attitude_protection : Saturate  UpperLimit=AP_ClimbRateLoop_MaxPitchCmdrad  LowerLimit=AP_ClimbRateLoop_MinPitchCmdrad
  theta_Cmd : Outport
  wires:
  climb_rate_mps/1 -> Sum/2, Scope2/2
  Sum1/1 -> pitch_attitude_protection/1
  AP_ClimbRateLoop_Ki/1 -> Discrete-Time Integrator/1
  Sum/1 -> AP_ClimbRateLoop_Ki/1, Subsystem/1(u)  "climb_rate_spdloop_error_mps"
  AP_ClimbRateLoop_Kp/1 -> ClimbRate_cmd_compare/2, Sum1/1
  Discrete-Time Integrator/1 -> Sum1/2, ClimbRate_cmd_compare/1
  climb_rate_cmd_spdloop/1 -> AP_ClimbRateLoop_ClimbRateCmdLPF/1, Scope2/3  "climb_rate_cmd_spdloop_mps"
  Angle Conversion/1 -> theta_Cmd/1, Scope/1  "theta_cmd_uncapped_deg"
  AP_ClimbRateLoop_ClimbRateCmdLPF/1 -> Sum/1, Scope2/1
  climb_rate_cmd_altloop_mps/1 -> Terminator/1
  Subsystem/1(y) -> AP_ClimbRateLoop_Kp/1
  pitch_attitude_protection/1 -> Angle Conversion/1

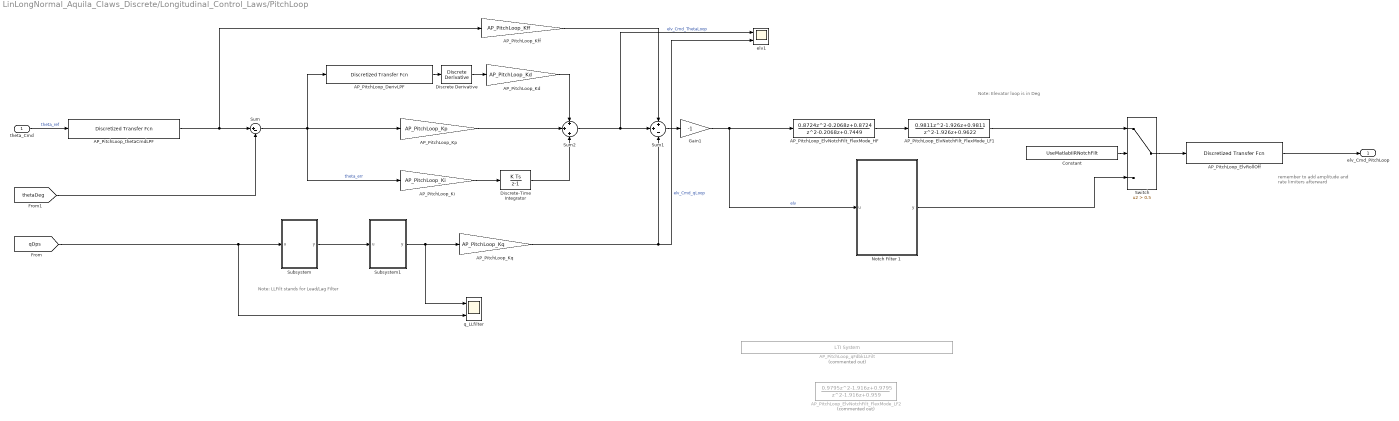
== system LinLongNormal_Aquila_Claws_Discrete/Longitudinal_Control_Laws/PitchLoop ==
  note: remember to add amplitude and
      | rate limiters afterward
  note: Note: Elevator loop is in Deg
  note: Note: LLFilt stands for Lead/Lag Filter
  theta_Cmd : Inport
  AP_PitchLoop_DerivLPF : discretizing/Discretized Transfer Fcn  Numerator=[1]  Denominator=[AP_PitchLoop_DerivLPFDenTau 1]  AbsTol=auto  SampleTime=0.04  method=zoh  Wc=1
  AP_PitchLoop_ElvNotchFilt_FlexMode_HF : DiscreteTransferFcn  Numerator=[0.8724 -0.2068 0.8724]  Denominator=[1 -0.2068 0.7449]  SampleTime=Ts
  AP_PitchLoop_ElvNotchFilt_FlexMode_LF1 : DiscreteTransferFcn  Numerator=[0.9811 -1.926 0.9811]  Denominator=[1 -1.926 0.9622]  SampleTime=Ts
  AP_PitchLoop_ElvNotchFilt_FlexMode_LF2 : DiscreteTransferFcn  Commented=on  Numerator=[0.9795 -1.916 0.9795]  Denominator=[1 -1.916 0.959]  SampleTime=Ts
  AP_PitchLoop_ElvRollOff : discretizing/Discretized Transfer Fcn  Numerator=[AP_PitchLoop_wn_ElvRollOff^2]  Denominator=[1 2*AP_PitchLoop_zeta_ElvRollOff*AP_PitchLoop_wn_ElvRollOff AP_PitchLoop_wn_ElvRollOff^2]  AbsTol=auto  SampleTime=0.04  method=zoh  Wc=1
  AP_PitchLoop_Kd : Gain  Gain=AP_PitchLoop_Kd
  AP_PitchLoop_Kff : Gain  Gain=AP_PitchLoop_Kff
  AP_PitchLoop_Ki : Gain  Gain=AP_PitchLoop_Ki
  AP_PitchLoop_Kp : Gain  Gain=AP_PitchLoop_Kp
  AP_PitchLoop_Kq : Gain  Gain=AP_PitchLoop_Kq
  AP_PitchLoop_qFdbkLLFilt : cstblocks/LTI System  Commented=on  sys=tf([1 AP_PitchLoop_qFdbkLLFiltNumCoe],[1 AP_PitchLoop_qFdbkLLFiltDenCoe])  IC=[]
  AP_PitchLoop_thetaCmdLPF : discretizing/Discretized Transfer Fcn  Numerator=[1]  Denominator=[AP_PitchLoop_thetaCmdLPFDenTau 1]  AbsTol=auto  SampleTime=0.04  method=zoh  Wc=1
  Constant : Constant  Value=UseMatlabIIRNotchFilt
  Discrete Derivative : simulink/Discrete/Discrete Derivative  gainval=1.0  ICPrevScaledInput=0.0  OutMin=[]  OutMax=[]  OutDataType=fixdt(1, 16)  OutScaling=2^-10  DoSatur=off
  Discrete-Time Integrator : DiscreteIntegrator  InitialConditionSetting=State (most efficient)  SampleTime=-1  ICPrevOutput=DiscIntNeverNeededParam  ICPrevScaledInput=DiscIntNeverNeededParam
  Gain1 : Gain  Gain=-1
  Notch Filter 1 : Subsystem
  Subsystem : Subsystem
  Subsystem1 : Subsystem
  Sum : Sum  Inputs=|+-
  Sum1 : Sum  Inputs=++-
  Sum2 : Sum  Inputs=+|+|+
  Switch : Switch  Criteria=u2 > Threshold  Threshold=0.5
  elv1 : Scope  NumInputPorts=2
  q_LLfilter : Scope  NumInputPorts=2
  elv_Cmd_PitchLoop : Outport
  wires:
  Sum/1 -> AP_PitchLoop_Kp/1, AP_PitchLoop_Ki/1, AP_PitchLoop_DerivLPF/1  "theta_err"
  AP_PitchLoop_Ki/1 -> Discrete-Time Integrator/1
  AP_PitchLoop_Kq/1 -> Sum1/3, elv1/2  "elv_Cmd_qLoop"
  AP_PitchLoop_Kff/1 -> Sum1/1
  [thetaDeg] -> Sum/2
  Sum2/1 -> Sum1/2, elv1/1  "elv_Cmd_ThetaLoop"
  Sum1/1 -> Gain1/1
  theta_Cmd/1 -> AP_PitchLoop_thetaCmdLPF/1  "theta_ref"
  AP_PitchLoop_ElvRollOff/1 -> elv_Cmd_PitchLoop/1
  Discrete Derivative/1 -> AP_PitchLoop_Kd/1
  AP_PitchLoop_DerivLPF/1 -> Discrete Derivative/1
  Discrete-Time Integrator/1 -> Sum2/3
  AP_PitchLoop_Kp/1 -> Sum2/2
  AP_PitchLoop_Kd/1 -> Sum2/1
  AP_PitchLoop_thetaCmdLPF/1 -> Sum/1, AP_PitchLoop_Kff/1
  Switch/1 -> AP_PitchLoop_ElvRollOff/1
  [qDps] -> q_LLfilter/2, Subsystem/1(u)
  Subsystem/1(y) -> Subsystem1/1(u)
  Gain1/1 -> AP_PitchLoop_ElvNotchFilt_FlexMode_HF/1, Notch Filter 1/1(u)  "elv"
  Notch Filter 1/1(y) -> Switch/3
  Constant/1 -> Switch/2
  AP_PitchLoop_ElvNotchFilt_FlexMode_HF/1 -> AP_PitchLoop_ElvNotchFilt_FlexMode_LF1/1
  Subsystem1/1(y) -> q_LLfilter/1, AP_PitchLoop_Kq/1
  AP_PitchLoop_ElvNotchFilt_FlexMode_LF1/1 -> Switch/1

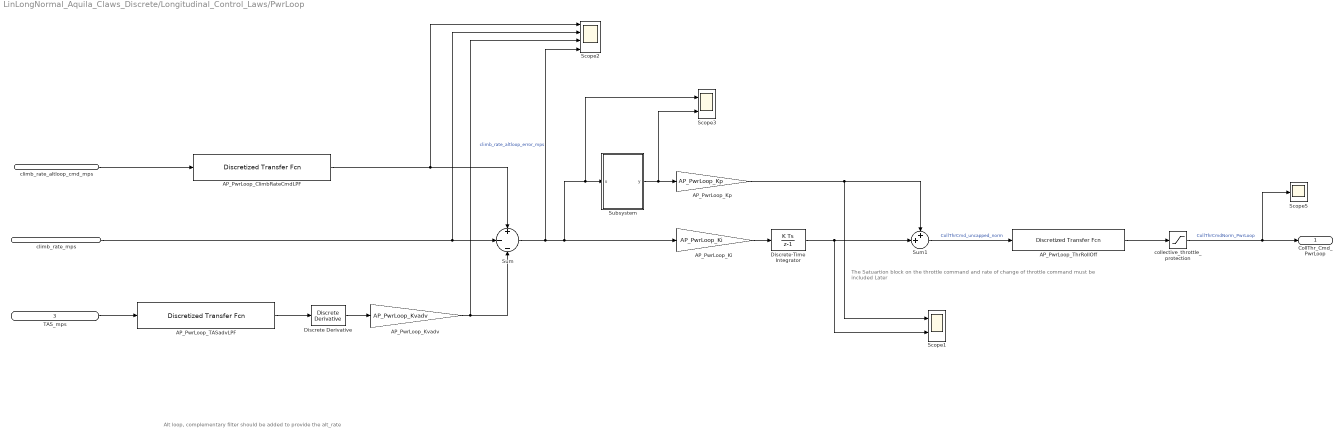
== system LinLongNormal_Aquila_Claws_Discrete/Longitudinal_Control_Laws/PwrLoop ==
  note: The Satuartion block on the throttle command and rate of change of throttle command must be
      | included Later
  note: Alt loop,
      | complementary filter should be added to provide the alt_rate
  climb_rate_altloop_cmd_mps : Inport
  climb_rate_mps : Inport  Port=2
  TAS_mps : Inport  Port=3
  AP_PwrLoop_ClimbRateCmdLPF : discretizing/Discretized Transfer Fcn  Numerator=[1]  Denominator=[AP_PwrLoop_ClimbRateCmdLPFDenTau 1]  AbsTol=auto  SampleTime=Ts  method=zoh  Wc=1
  AP_PwrLoop_Ki : Gain  Gain=AP_PwrLoop_Ki
  AP_PwrLoop_Kp : Gain  Gain=AP_PwrLoop_Kp
  AP_PwrLoop_Kvadv : Gain  Gain=AP_PwrLoop_Kvadv
  AP_PwrLoop_TASadvLPF : discretizing/Discretized Transfer Fcn  Numerator=[1]  Denominator=[AP_TASLoop_TASadvLPFDenTau 1]  AbsTol=auto  SampleTime=Ts  method=zoh  Wc=1
  AP_PwrLoop_ThrRollOff : discretizing/Discretized Transfer Fcn  Numerator=[AP_PwrLoop_wn_ThrRollOff^2]  Denominator=[1 2*AP_PwrLoop_zeta_ThrRollOff*AP_PwrLoop_wn_ThrRollOff AP_PwrLoop_wn_ThrRollOff^2]  AbsTol=auto  SampleTime=0.04  method=zoh  Wc=1
  Discrete Derivative : simulink/Discrete/Discrete Derivative  gainval=1.0  ICPrevScaledInput=0.0  OutMin=[]  OutMax=[]  OutDataType=fixdt(1, 16)  OutScaling=2^-10  DoSatur=off
  Discrete-Time Integrator : DiscreteIntegrator  InitialConditionSetting=State (most efficient)  SampleTime=-1  LimitOutput=on  UpperSaturationLimit=0.15  LowerSaturationLimit=-0.15  ICPrevOutput=DiscIntNeverNeededParam  ICPrevScaledInput=DiscIntNeverNeededParam
  Scope1 : Scope  NumInputPorts=2
  Scope2 : Scope  NumInputPorts=4
  Scope3 : Scope  NumInputPorts=2
  Scope5 : Scope
  Subsystem : Subsystem
  Sum : Sum  Inputs=+|-|-
  Sum1 : Sum  Inputs=++|
  collective_throttle_protection : Saturate  UpperLimit=AP_PwrLoop_MaxThrCmdNorm  LowerLimit=AP_PwrLoop_MinThrCmdNorm
  CollThr_Cmd_PwrLoop : Outport
  wires:
  AP_PwrLoop_Ki/1 -> Discrete-Time Integrator/1
  Sum/1 -> Scope2/4, AP_PwrLoop_Ki/1, Scope3/1, Subsystem/1(u)  "climb_rate_altloop_error_mps"
  AP_PwrLoop_Kp/1 -> Sum1/1, Scope1/1
  Discrete-Time Integrator/1 -> Sum1/2, Scope1/2
  climb_rate_altloop_cmd_mps/1 -> AP_PwrLoop_ClimbRateCmdLPF/1
  AP_PwrLoop_ClimbRateCmdLPF/1 -> Scope2/1, Sum/1
  climb_rate_mps/1 -> Scope2/2, Sum/2
  Sum1/1 -> AP_PwrLoop_ThrRollOff/1  "CollThrCmd_uncapped_norm"
  AP_PwrLoop_TASadvLPF/1 -> Discrete Derivative/1
  Discrete Derivative/1 -> AP_PwrLoop_Kvadv/1
  TAS_mps/1 -> AP_PwrLoop_TASadvLPF/1
  AP_PwrLoop_Kvadv/1 -> Scope2/3, Sum/3
  collective_throttle_protection/1 -> Scope5/1, CollThr_Cmd_PwrLoop/1  "CollThrCmdNorm_PwrLoop"
  AP_PwrLoop_ThrRollOff/1 -> collective_throttle_protection/1
  Subsystem/1(y) -> AP_PwrLoop_Kp/1, Scope3/2
